simulink model "behavior_fsm"  (R2026a)
settings: Solver=FixedStepDiscrete  FixedStep=0.1
settings Model: Creator=Lenovo  LastModifiedBy=Lenovo

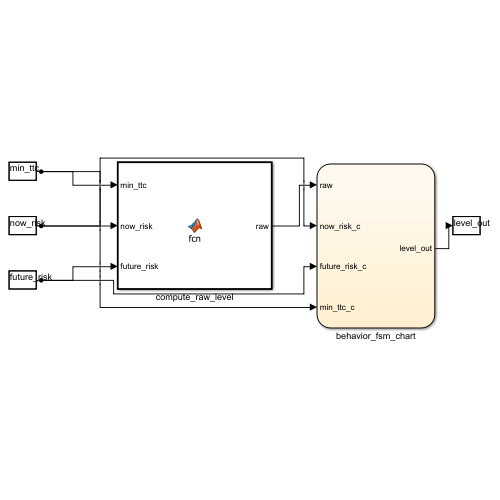
[thumbnail: Simulink's stored preview of the top-level diagram]
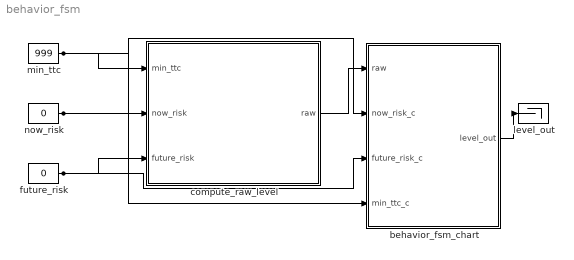
== system behavior_fsm ==
  behavior_fsm_chart : Stateflow chart  TreatAsAtomicUnit=on
  compute_raw_level : MATLAB Function  TreatAsAtomicUnit=on
  future_risk : Constant  Value=0
  level_out : Terminator
  min_ttc : Constant  Value=999
  now_risk : Constant  Value=0
  wires:
  min_ttc/1 -> compute_raw_level/1(min_ttc), behavior_fsm_chart/4(min_ttc_c)
  now_risk/1 -> compute_raw_level/2(now_risk), behavior_fsm_chart/2(now_risk_c)
  future_risk/1 -> compute_raw_level/3(future_risk), behavior_fsm_chart/3(future_risk_c)
  compute_raw_level/1(raw) -> behavior_fsm_chart/1(raw)
  behavior_fsm_chart/1(level_out) -> level_out/1

== matlab function behavior_fsm/compute_raw_level ==
  data: min_ttc input; raw output; now_risk input; future_risk input
function raw = compute_raw_level(min_ttc, now_risk, future_risk)     
                                                                    % Direct transliteration of M5_Pipeline/fsm.py's _raw_level -- branch
                                                                    % ORDER matters (AVOID-before-YIELD live-incident fix, see fsm.py's  
                                                                    % own docstring/README for why). RED=3, YELLOW=2, GREEN=1, NONE=0.   
                                                                    TTC_EMERGENCY_S = 1.5;                                               
                                                                    TTC_AVOID_S = 4.0;                                                   
                                                                    TTC_FOLLOW_S = 8.0;                                                  
                                                                    RED = 3; YELLOW = 2;                                                 
                                                                                                                                         
                                                                    if min_ttc <= TTC_EMERGENCY_S                                        
                                                                        raw = 4; return;                                                 
                                                                    end                                                                  
                                                                    if now_risk == RED                                                   
                                                                        raw = 4; return;                                                 
                                                                    end                                                                  
                                                                    if min_ttc <= TTC_AVOID_S                                            
                                                                        raw = 2; return;                                                 
                                                                    end                                                                  
                                                                    if now_risk == RED || now_risk == YELLOW                             
                                                                        raw = 2; return;                                                 
                                                                    end                                                                  
                                                                    if future_risk == RED || future_risk == YELLOW                       
                                                                        raw = 3; return;                                                 
                                                                    end                                                                  
                                                                    if min_ttc <= TTC_FOLLOW_S                                           
                                                                        raw = 1; return;                                                 
                                                                    end                                                                  
                                                                    raw = 0;                                                             
                                                                    end

== stateflow chart behavior_fsm/behavior_fsm_chart ==
  state CRUISE
    entry: level_out = 0;
  state FOLLOW
    entry: level_out = 1;
  state AVOID
    entry: level_out = 2;
  state YIELD
    entry: level_out = 3;
  state EMERGENCY_BRAKE
    entry: level_out = 4;
  FOLLOW -> CRUISE [order 4] : [(raw == 0) && (min_ttc_c > 8.0 + 0.5)]
  YIELD -> CRUISE [order 2] : [(raw == 0) && (future_risk_c == 0)]
  (default) -> CRUISE
  EMERGENCY_BRAKE -> CRUISE [order 1] : [(raw == 0) && (min_ttc_c > 1.5 + 0.5) && (now_risk_c ~= 3)]
  AVOID -> CRUISE [order 3] : [(raw == 0) && (min_ttc_c > 4.0 + 0.5) && (now_risk_c == 0)]
  FOLLOW -> AVOID [order 1] : [raw == 2]
  AVOID -> FOLLOW [order 4] : [(raw == 1) && (min_ttc_c > 4.0 + 0.5) && (now_risk_c == 0)]
  CRUISE -> FOLLOW [order 1] : [raw == 1]
  EMERGENCY_BRAKE -> FOLLOW [order 2] : [(raw == 1) && (min_ttc_c > 1.5 + 0.5) && (now_risk_c ~= 3)]
  YIELD -> FOLLOW [order 3] : [(raw == 1) && (future_risk_c == 0)]
  FOLLOW -> EMERGENCY_BRAKE [order 3] : [raw == 4]
  CRUISE -> EMERGENCY_BRAKE [order 4] : [raw == 4]
  YIELD -> AVOID [order 4] : [(raw == 2) && (future_risk_c == 0)]
  CRUISE -> YIELD [order 3] : [raw == 3]
  CRUISE -> AVOID [order 2] : [raw == 2]
  FOLLOW -> YIELD [order 2] : [raw == 3]
  EMERGENCY_BRAKE -> AVOID [order 3] : [(raw == 2) && (min_ttc_c > 1.5 + 0.5) && (now_risk_c ~= 3)]
  AVOID -> YIELD [order 1] : [raw == 3]
  EMERGENCY_BRAKE -> YIELD [order 4] : [(raw == 3) && (min_ttc_c > 1.5 + 0.5) && (now_risk_c ~= 3)]
  YIELD -> EMERGENCY_BRAKE [order 1] : [raw == 4]
  AVOID -> EMERGENCY_BRAKE [order 2] : [raw == 4]
  data: raw input double; now_risk_c input double; future_risk_c input double; min_ttc_c input double; level_out output double
